simulink model "ControllerSelector"  (R2024a)
settings: Solver=VariableStepAuto  StartTime=0.0  StopTime=tsReplan*2  FixedStep=0.001  RelTol=1e-3
undefined symbols (not defined in the file or in its folder): tsIntegrator
settings Model: DataDictionary=PlannerData.sldd  Creator=cstabile  LastModifiedBy=cstabile
settings DataIOCC: SaveOutput=off  SaveTime=off
settings SFSimCC: SimTargetLang=C++
settings RTWCC: GPUComputeCapability=3.5

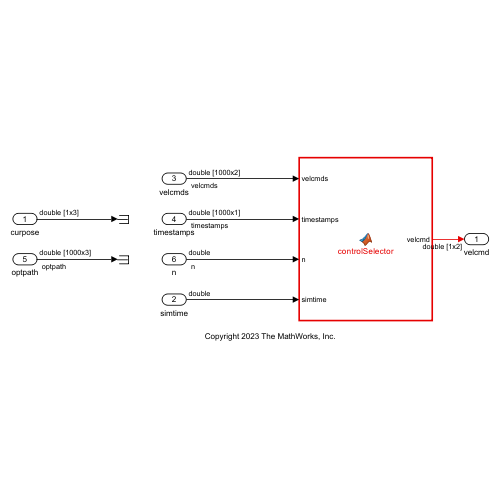
[thumbnail: Simulink's stored preview of the top-level diagram]
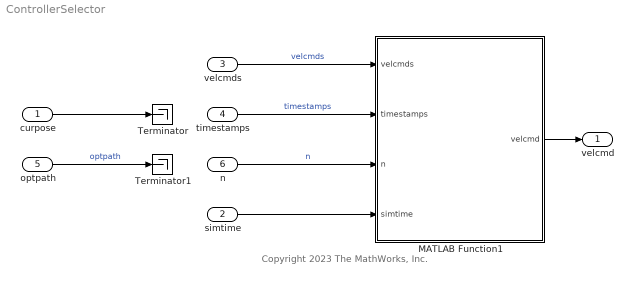
== system ControllerSelector ==
  note: Copyright 2023 The MathWorks, Inc.
  curpose : Inport  OutDataTypeStr=double  PortDimensions=[1 3]
  simtime : Inport  Port=2  OutDataTypeStr=double  PortDimensions=1  SampleTime=tsIntegrator
  velcmds : Inport  Port=3  OutDataTypeStr=double  PortDimensions=[1000 2]  SampleTime=tsIntegrator
  timestamps : Inport  Port=4  OutDataTypeStr=double  PortDimensions=[1000 1]  SampleTime=tsIntegrator
  optpath : Inport  Port=5  OutDataTypeStr=double  PortDimensions=[1000 3]
  n : Inport  Port=6  OutDataTypeStr=double  PortDimensions=1  SampleTime=tsIntegrator
  MATLAB Function1 : MATLAB Function  TreatAsAtomicUnit=on
  Terminator : Terminator
  Terminator1 : Terminator
  velcmd : Outport  OutDataTypeStr=double  PortDimensions=[1 2]  SampleTime=tsIntegrator
  wires:
  optpath/1 -> Terminator1/1  "optpath"
  curpose/1 -> Terminator/1
  MATLAB Function1/1(velcmd) -> velcmd/1
  simtime/1 -> MATLAB Function1/4(simtime)
  timestamps/1 -> MATLAB Function1/2(timestamps)  "timestamps"
  n/1 -> MATLAB Function1/3(n)  "n"
  velcmds/1 -> MATLAB Function1/1(velcmds)  "velcmds"

== matlab function ControllerSelector/MATLAB Function1 ==
  settings: updateMethod=DISCRETE  sampleTime=tsIntegrator
  data: velcmds input; velcmd output size=[1 2]; timestamps input; n input; simtime input
function velcmd = controlSelector(velcmds, timestamps, n, simtime)
    velcmd_ = velocityCommand(velcmds(1:n,:), timestamps(1:n,:), simtime);
    velcmd = velcmd_(1,1:2);
